simulink model "torqueFree"  (R2022a)
settings: Solver=VariableStepAuto  StartTime=0.0  StopTime=6000  RelTol=1e-3
values from neighbouring files (symbols this model uses):
  I = ImatGlo    [TorqueFreeMotion.m]    (also in torqueFreeCaller.m = diag(nominal.moi))
  T = [0;0;0]    [TorqueFreeMotion.m]    (also in torqueFreeCaller.m)
  X0 = [w0;E0;eps0;eta0]    [TorqueFreeMotion.m]    (also in torqueFreeCaller.m)
settings Model: Creator=Josh2  LastModifiedBy=Josh2

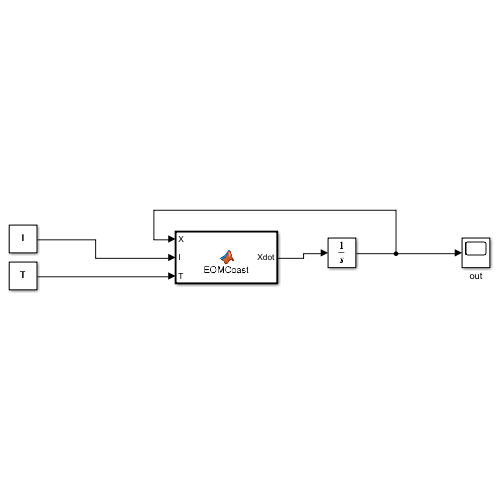
[thumbnail: Simulink's stored preview of the top-level diagram]
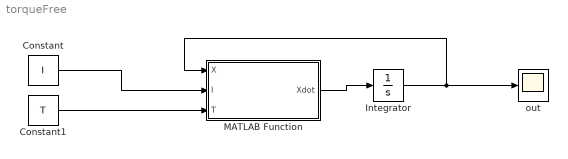
== system torqueFree ==
  Constant : Constant  Value=I
  Constant1 : Constant  Value=T
  Integrator : Integrator  InitialCondition=X0
  MATLAB Function : MATLAB Function  TreatAsAtomicUnit=on
  out : Scope
  wires:
  MATLAB Function/1(Xdot) -> Integrator/1
  Integrator/1 -> MATLAB Function/1(X), out/1
  Constant/1 -> MATLAB Function/2(I)
  Constant1/1 -> MATLAB Function/3(T)

== matlab function torqueFree/MATLAB Function ==
  data: Xdot output; X input; I input; T input
function Xdot = EOMCoast(X,I,T)
% % global ImatGlo
% % 
% % I = ImatGlo;
% 
% I = load("C:\AERO421\FinalProj\MOI.mat");
% I = I.moi;
% I = diag(I);
% % I = [812.03958333333,0,0
% % 0,545.372916666667,0
% % 0,0,627.708333333333];

w = X(1:3);
E = X(4:6);
eps = X(7:9);
eta = X(10);
% T = [0;0;0]; % torque


Cx = @(theta)...
    [[1 0 0];...
    [0 cos(theta) sin(theta)];...
    [0 -sin(theta) cos(theta)]];

Cy = @(theta)...
    [[cos(theta) 0 -sin(theta)];...
    [ 0 1 0];...
    [sin(theta) 0 cos(theta)]];

Cz = @(theta)...
    [[cos(theta) sin(theta) 0];...
    [-sin(theta) cos(theta) 0];...
    [0 0 1]];

mat = Cx(E(3))*Cy(E(2))*Cz(E(1));
Edot = mat*w;

epsx = cross(eps);
epsdot = .5*(eta*eye(3)+epsx)*w;
etadot = -.5*eps'*w;

wx = cross(w);
wdot = -inv(I)*(wx*I*w-T);

Xdot = [wdot;Edot;epsdot;etadot];

% because simulink sucks, I have to remove argument validation from my
% cross function. Below is percicely that
    function mx = cross(m)
        mx = zeros(3);
        mx(1,2) = -m(3);
        mx(1,3) =  m(2);
        mx(2,3) = -m(1);

        mx(2,1) =  m(3);
        mx(3,1) = -m(2);
        mx(3,2) =  m(1);
    end

end
